simulink model "Model_2_1"  (R2024a)
settings: Solver=ode15s  StartTime=0.0  StopTime=100  FixedStep=0.0001  MaxStep=0.01  RelTol=1e-3  AbsTol=1e-3  EnableMultiTasking=on
model workspace (MATLAB code in the model file):
  | F_load_x= 0;   %[N]
  | F_load_y=-1e4; %[N]
  | 
  | d=0.01;   %[m]
  | l=1;      %[m]
  | L=l;      %[m] Node distance
  | H=l;      %[m] Node distance
  | Density=7800; %[kg/m^3]
  | E=210;   %[GPa]
  | G=79;    %[GPa]
  | bm=0.01; %[1/s] Default
  | bk=0.01; %[s] Default
  | 
  | b_rj=1; %[N*m*s/rad] Damp.Coef.Revolut joints
  | 
  | Size_frame=30; %[pixel]
undefined symbols (not defined in the file): F_x, F_y, X, Y, Z
libraries: sm_lib x173, nesl_utility x36, fl_lib x6, simulink x1
(part 1 of 5)
settings Model: NumberOfSteps=100000  Creator=Ing. Štefan Ondočko  LastModifiedBy=Ing. Štefan Ondočko
settings SolverCC: AutoScaleAbsTol=off  MaxZcPerStep=1
settings DataIOCC: LimitDataPoints=on  MaxDataPoints=10000  ReturnWorkspaceOutputs=off
settings OptimizationCC: ReuseModelBlockBuffer=off  LifeSpan=inf
settings DebuggingCC: UnconnectedInputMsg=warning  UnconnectedOutputMsg=warning  UnconnectedLineMsg=warning  AllowSymbolicDim=off  SubsystemReferenceDiagnosticForUnitTest=warning  SFUnexpectedBacktrackingDiag=warning  SFNoUnconditionalDefaultTransitionDiag=warning  SFExecutionAtInitializationDiag=none  ArithmeticOperatorsInVariantConditions=warning
settings ModelReferenceCC: EnableRefExpFcnMdlSchedulingChecks=on
settings SFSimCC: SimUseLocalCustomCode=off  CustomCodeUndefinedFunction=UseInterfaceOnly
settings RTWCC: RTWUseLocalCustomCode=off  GPUComputeCapability=3.5  DLArmComputeVersion=19.05
settings CodeAppCC: StateflowObjectComments=on
settings GRTTargetCC: TargetLangStandard=C89/C90 (ANSI)
settings ConfigComp: CovMetricSettings=dw  CovSaveCumulativeToWorkspaceVar=on  CovSaveSingleToWorkspaceVar=on  CovExternalEMLEnable=off  CovSFcnEnable=off
settings SimscapeCC: SimscapeLogType=all  SimscapeLogSimulationStatistics=on  SimscapeLogDataHistory=10000
settings ExplorerConfigSet: InternalSimMechanicsExplorerSettings="<ExplorerConfiguration><canonicalview>default</canonicalview><AnimationSetting><BasePlaybackSpeed>1.0</BasePlaybackSpeed><PlaybackSpeedFactor>2.0</PlaybackSpeedFactor></AnimationSetting><TilePanel><TileInfo><Tiles Columns=\"1\" Count=\"1\" Rows=\"1\"><Column Weight=\"1\"/><Row Weight=\"1\"/><Tile Height=\"1\" Width=\"1\" X=\"0\" Y=\"0\"/></Tiles></TileInfo><SceneInfo><SceneViewer><BGColor><R>1</R><G>1</G><B>1</B></BGColor><Camera><DoPerspective>off</DoPerspective><Position><X>1.34160017439744395</X><Y>2.43472426416735921</Y><Z>3.19868175252832421</Z></Position><Center><X>1.34160017439744395</X><Y>2.43472426416735921</Y><Z>1.1802899990698279e-08</Z></Center><Up><X>0</X><Y>1</Y><Z>-0</Z></Up><ViewLimDist>1</ViewLimDist><YLim>3.18022072065698147</YLim><XLim>1.97030216076793452</XLim></Camera></SceneViewer></SceneInfo></TilePanel><MechEditorPanel><Cameras/><GfxPanelCameraMap/><VideoCreator><PlaybackSpeedRatio>1.0</PlaybackSpeedRatio><FrameRate>30</FrameRate><VideoFormat>Motion JPEG AVI</VideoFormat><FrameSize>auto</FrameSize></VideoCreator></MechEditorPanel></ExplorerConfiguration>"

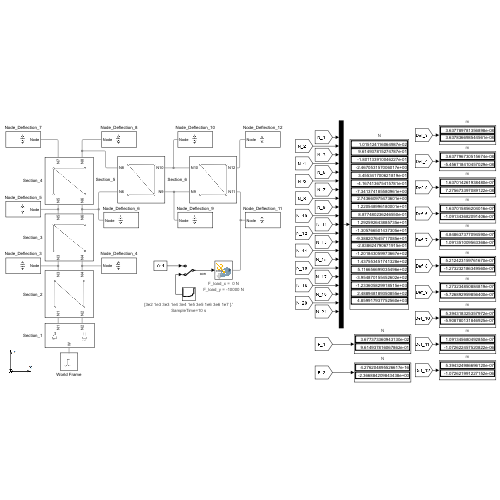
[thumbnail: Simulink's stored preview of the top-level diagram]
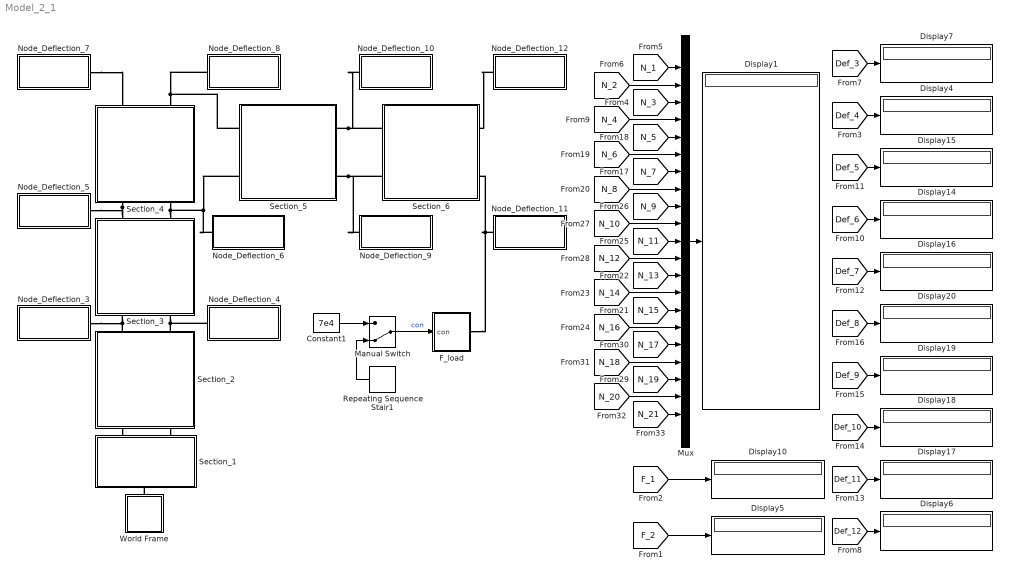
== system Model_2_1 ==
  Constant1 : Constant  Value=7e4
  Display{1,4..7,10,14..20} (13 alike) : Display
      Display1 settings: Description=N  AttributesFormatString=%<Description>  Format=long_e
      Display10 settings: Description=N  AttributesFormatString=%<Description>  Format=long_e
      Display14 settings: Description=m  AttributesFormatString=%<Description>  Format=long_e
      Display15 settings: Description=m  AttributesFormatString=%<Description>  Format=long_e
      Display16 settings: Description=m  AttributesFormatString=%<Description>  Format=long_e
      Display17 settings: Description=m  AttributesFormatString=%<Description>  Format=long_e
      Display18 settings: Description=m  AttributesFormatString=%<Description>  Format=long_e
      Display19 settings: Description=m  AttributesFormatString=%<Description>  Format=long_e
      Display20 settings: Description=m  AttributesFormatString=%<Description>  Format=long_e
      Display4 settings: Description=m  AttributesFormatString=%<Description>  Format=long_e
      Display5 settings: Description=N  AttributesFormatString=%<Description>  Format=long_e
      Display6 settings: Description=m  AttributesFormatString=%<Description>  Format=long_e
      Display7 settings: Description=m  AttributesFormatString=%<Description>  Format=long_e
  F_load : Subsystem  mask{Fx=F_load_x, Fy=F_load_y, F=norm([F_x F_y])}
      mask prompts: Fx "Load Fx (N)"; Fy "Load Fy (N)"; F "Load F (N)"
      settings: AttributesFormatString=|
      | %<Fx> =  0 N
      | %<Fy> = -10000 N
      mask Display: image('D:sila_F.png');
  Manual Switch : ManualSwitch  CurrentSetting=0
  Mux : Mux  Inputs=21
  Node_Deflection_10 : Subsystem
  Node_Deflection_11 : Subsystem
  Node_Deflection_12 : Subsystem
  Node_Deflection_3 : Subsystem
  Node_Deflection_4 : Subsystem
  Node_Deflection_5 : Subsystem
  Node_Deflection_6 : Subsystem
  Node_Deflection_7 : Subsystem
  Node_Deflection_8 : Subsystem
  Node_Deflection_9 : Subsystem
  Repeating Sequence Stair1 : simulink/Sources/Repeating Sequence Stair  OutValues=[3e2 1e3 3e3 1e4 3e4 1e5 3e5 1e6 3e6 1e7 ].'  tsamp=10  OutMin=[]  OutMax=[]  OutDataTypeStr=double  OutputDataTypeScalingMode=double  OutDataType=fixdt(0,8)  ConRadixGroup=Best Precision: Vector-wise  OutScaling=2^-12
      settings: AttributesFormatString=|
      | %<OutValues>
      | SampleTime=%<tsamp> s
  Section_1 : Subsystem
      settings: PortSchema="{\"entries\":[{\"content\":{\"sides\":[{\"content\":{},\"type\":\"ConnectorPlacement.EquallySpacedRectSide\",\"uuid\":\"639cab07-c461-4b38-814c-b2f66736f8dc\"},{\"content\":{\"side\":\"RIGHT\"},\"type\":\"ConnectorPlacement.EquallySpacedRectSide\",\"uuid\":\"511a9213-a72f-4349-881c-c7bf2be19ca2\"},{\"content\":{\"connectorIds\":[\"LConn1\"],\"side\":\"TOP\"},\"type\":\"ConnectorPlacement.EquallySpacedRectSide\",\"uuid\":\"5e8f2857-f7f3-429a-845e-93ee7ceff152\"},{\"content\":{\"connectorIds\":[\"RConn1\",\"RConn2\"],\"side\":\"BOTTOM\"},\"type\":\"ConnectorPlacement.EquallySpacedRectSide\",\"uuid\":\"39b416cf-f84e-45de-8d0c-fe880f5852f0\"}]},\"type\":\"ConnectorPlacement.EquallySpacedConnector\",\"uuid\":\"63df7647-7376-4d28-81b8-bff3ff006582\"}],\"packageUris\":[\"http://schema.mathworks.com/mf0/Connector/R2020b\"],\"version\":\"1.0\"}"
  Section_2 : Subsystem
      settings: PortSchema="{\"entries\":[{\"content\":{\"sides\":[{\"content\":{},\"type\":\"ConnectorPlacement.EquallySpacedRectSide\",\"uuid\":\"9852856a-cfaf-4274-b31b-57367341680d\"},{\"content\":{\"side\":\"RIGHT\"},\"type\":\"ConnectorPlacement.EquallySpacedRectSide\",\"uuid\":\"3ac774e0-1e79-4574-83fc-c3ad9c08ab46\"},{\"content\":{\"connectorIds\":[\"LConn1\",\"LConn2\"],\"side\":\"TOP\"},\"type\":\"ConnectorPlacement.EquallySpacedRectSide\",\"uuid\":\"0b881cdb-833a-4bc4-a75d-99faa647454f\"},{\"content\":{\"connectorIds\":[\"RConn1\",\"RConn2\"],\"side\":\"BOTTOM\"},\"type\":\"ConnectorPlacement.EquallySpacedRectSide\",\"uuid\":\"d5c54b3f-7996-4e81-879d-4e982bdffaf2\"}]},\"type\":\"ConnectorPlacement.EquallySpacedConnector\",\"uuid\":\"66ee5201-3e9b-4b60-9348-bbbcd71d5871\"}],\"packageUris\":[\"http://schema.mathworks.com/mf0/Connector/R2020b\"],\"version\":\"1.0\"}"
  Section_3 : Subsystem
      settings: PortSchema="{\"entries\":[{\"content\":{\"sides\":[{\"content\":{},\"type\":\"ConnectorPlacement.EquallySpacedRectSide\",\"uuid\":\"9852856a-cfaf-4274-b31b-57367341680d\"},{\"content\":{\"side\":\"RIGHT\"},\"type\":\"ConnectorPlacement.EquallySpacedRectSide\",\"uuid\":\"3ac774e0-1e79-4574-83fc-c3ad9c08ab46\"},{\"content\":{\"connectorIds\":[\"LConn1\",\"LConn2\"],\"side\":\"TOP\"},\"type\":\"ConnectorPlacement.EquallySpacedRectSide\",\"uuid\":\"0b881cdb-833a-4bc4-a75d-99faa647454f\"},{\"content\":{\"connectorIds\":[\"RConn1\",\"RConn2\"],\"side\":\"BOTTOM\"},\"type\":\"ConnectorPlacement.EquallySpacedRectSide\",\"uuid\":\"d5c54b3f-7996-4e81-879d-4e982bdffaf2\"}]},\"type\":\"ConnectorPlacement.EquallySpacedConnector\",\"uuid\":\"66ee5201-3e9b-4b60-9348-bbbcd71d5871\"}],\"packageUris\":[\"http://schema.mathworks.com/mf0/Connector/R2020b\"],\"version\":\"1.0\"}"
  Section_4 : Subsystem
      settings: PortSchema="{\"entries\":[{\"content\":{\"sides\":[{\"content\":{},\"type\":\"ConnectorPlacement.EquallySpacedRectSide\",\"uuid\":\"9852856a-cfaf-4274-b31b-57367341680d\"},{\"content\":{\"side\":\"RIGHT\"},\"type\":\"ConnectorPlacement.EquallySpacedRectSide\",\"uuid\":\"3ac774e0-1e79-4574-83fc-c3ad9c08ab46\"},{\"content\":{\"connectorIds\":[\"LConn1\",\"LConn2\"],\"side\":\"TOP\"},\"type\":\"ConnectorPlacement.EquallySpacedRectSide\",\"uuid\":\"0b881cdb-833a-4bc4-a75d-99faa647454f\"},{\"content\":{\"connectorIds\":[\"RConn1\",\"RConn2\"],\"side\":\"BOTTOM\"},\"type\":\"ConnectorPlacement.EquallySpacedRectSide\",\"uuid\":\"d5c54b3f-7996-4e81-879d-4e982bdffaf2\"}]},\"type\":\"ConnectorPlacement.EquallySpacedConnector\",\"uuid\":\"66ee5201-3e9b-4b60-9348-bbbcd71d5871\"}],\"packageUris\":[\"http://schema.mathworks.com/mf0/Connector/R2020b\"],\"version\":\"1.0\"}"
  Section_5 : Subsystem
      settings: PortSchema="{\"entries\":[{\"content\":{\"sides\":[{\"content\":{},\"type\":\"ConnectorPlacement.EquallySpacedRectSide\",\"uuid\":\"9852856a-cfaf-4274-b31b-57367341680d\"},{\"content\":{\"side\":\"RIGHT\"},\"type\":\"ConnectorPlacement.EquallySpacedRectSide\",\"uuid\":\"3ac774e0-1e79-4574-83fc-c3ad9c08ab46\"},{\"content\":{\"connectorIds\":[\"LConn1\",\"LConn2\"],\"side\":\"TOP\"},\"type\":\"ConnectorPlacement.EquallySpacedRectSide\",\"uuid\":\"0b881cdb-833a-4bc4-a75d-99faa647454f\"},{\"content\":{\"connectorIds\":[\"RConn1\",\"RConn2\"],\"side\":\"BOTTOM\"},\"type\":\"ConnectorPlacement.EquallySpacedRectSide\",\"uuid\":\"d5c54b3f-7996-4e81-879d-4e982bdffaf2\"}]},\"type\":\"ConnectorPlacement.EquallySpacedConnector\",\"uuid\":\"66ee5201-3e9b-4b60-9348-bbbcd71d5871\"}],\"packageUris\":[\"http://schema.mathworks.com/mf0/Connector/R2020b\"],\"version\":\"1.0\"}"
  Section_6 : Subsystem
      settings: PortSchema="{\"entries\":[{\"content\":{\"sides\":[{\"content\":{},\"type\":\"ConnectorPlacement.EquallySpacedRectSide\",\"uuid\":\"9852856a-cfaf-4274-b31b-57367341680d\"},{\"content\":{\"side\":\"RIGHT\"},\"type\":\"ConnectorPlacement.EquallySpacedRectSide\",\"uuid\":\"3ac774e0-1e79-4574-83fc-c3ad9c08ab46\"},{\"content\":{\"connectorIds\":[\"LConn1\",\"LConn2\"],\"side\":\"TOP\"},\"type\":\"ConnectorPlacement.EquallySpacedRectSide\",\"uuid\":\"0b881cdb-833a-4bc4-a75d-99faa647454f\"},{\"content\":{\"connectorIds\":[\"RConn1\",\"RConn2\"],\"side\":\"BOTTOM\"},\"type\":\"ConnectorPlacement.EquallySpacedRectSide\",\"uuid\":\"d5c54b3f-7996-4e81-879d-4e982bdffaf2\"}]},\"type\":\"ConnectorPlacement.EquallySpacedConnector\",\"uuid\":\"66ee5201-3e9b-4b60-9348-bbbcd71d5871\"}],\"packageUris\":[\"http://schema.mathworks.com/mf0/Connector/R2020b\"],\"version\":\"1.0\"}"
  World Frame : Subsystem
      settings: PortSchema="{\"entries\":[{\"content\":{\"sides\":[{\"content\":{},\"type\":\"ConnectorPlacement.EquallySpacedRectSide\",\"uuid\":\"6a8e21d3-b0b2-4758-a6c8-a7be5ecb73b9\"},{\"content\":{\"side\":\"RIGHT\"},\"type\":\"ConnectorPlacement.EquallySpacedRectSide\",\"uuid\":\"42798d98-bef9-4838-9935-056c1ef1235d\"},{\"content\":{\"connectorIds\":[\"LConn1\"],\"side\":\"TOP\"},\"type\":\"ConnectorPlacement.EquallySpacedRectSide\",\"uuid\":\"7c8f84cf-9fc0-4b00-b00b-766e511bcfac\"}]},\"type\":\"ConnectorPlacement.EquallySpacedConnector\",\"uuid\":\"93a5f294-2ff9-4ffa-a830-6e6e0d522148\"}],\"packageUris\":[\"http://schema.mathworks.com/mf0/Connector/R2020b\"],\"version\":\"1.0\"}"
  wires:
  Constant1/1 -> Manual Switch/1
  Manual Switch/1 -> F_load/1(con)  "con"
  [N_21] -> Mux/21
  Mux/1 -> Display1/1
  [N_20] -> Mux/20
  [N_18] -> Mux/18
  [N_16] -> Mux/16
  [N_12] -> Mux/12
  [N_5] -> Mux/5
  [N_10] -> Mux/10
  [N_4] -> Mux/4
  [N_2] -> Mux/2
  [N_17] -> Mux/17
  [N_19] -> Mux/19
  [N_15] -> Mux/15
  [Def_6] -> Display14/1
  [N_11] -> Mux/11
  [N_9] -> Mux/9
  [Def_9] -> Display19/1
  [N_7] -> Mux/7
  [Def_8] -> Display20/1
  [N_8] -> Mux/8
  [Def_11] -> Display17/1
  [N_1] -> Mux/1
  [N_14] -> Mux/14
  [Def_5] -> Display15/1
  [Def_7] -> Display16/1
  [N_3] -> Mux/3
  [N_6] -> Mux/6
  [Def_3] -> Display7/1
  [Def_10] -> Display18/1
  [N_13] -> Mux/13
  Repeating Sequence Stair1/1 -> Manual Switch/2
  [F_1] -> Display10/1
  [F_2] -> Display5/1
  [Def_12] -> Display6/1
  [Def_4] -> Display4/1
  connections:
  Node_Deflection_4/LConn1 -- Section_2/RConn2 -- Section_3/LConn2
  Node_Deflection_11/LConn1 -- F_load/RConn1 -- Section_6/LConn1
  Section_5/LConn1 -- Section_6/RConn1 -- Node_Deflection_9/LConn1
  Section_5/RConn1 -- Section_4/LConn2 -- Section_3/RConn2 -- Node_Deflection_6/LConn1
  Section_4/RConn2 -- Section_5/RConn2 -- Node_Deflection_8/LConn1
  Node_Deflection_3/LConn1 -- Section_2/RConn1 -- Section_3/LConn1
  Section_5/LConn2 -- Section_6/RConn2 -- Node_Deflection_10/LConn1
  Section_3/RConn1 -- Section_4/LConn1 -- Node_Deflection_5/LConn1
  Node_Deflection_12/LConn1 -- Section_6/LConn2
  Node_Deflection_7/LConn1 -- Section_4/RConn1
  World Frame/LConn1 -- Section_1/LConn1
  Section_2/LConn2 -- Section_1/RConn2
  Section_2/LConn1 -- Section_1/RConn1

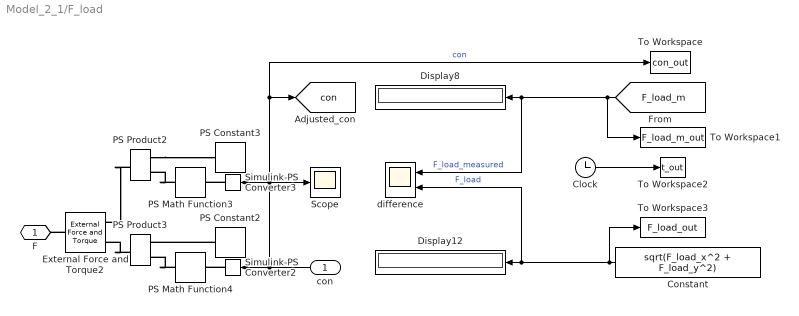
== system Model_2_1/F_load ==
  con : Inport
  Clock : Clock
  Constant : Constant  Value=sqrt(F_load_x^2 + F_load_y^2)
  Display12 : Display
      settings: Description=N  AttributesFormatString=%<Description>  Format=long_e
  Display8 : Display
      settings: Description=N  AttributesFormatString=%<Description>  Format=long_e
  External Force and Torque2 : sm_lib/Forces and Torques/External Force and Torque  EnableForceX=on  EnableForceY=on  EnableForceZ=off  EnableForce=off  ForceResolutionFrame=World  EnableTorqueX=off  EnableTorqueY=off  EnableTorqueZ=off  EnableTorque=off  TorqueResolutionFrame=AttachedFrame
  PS Constant2 : fl_lib/Physical Signals/Sources/PS Constant  constant=F_load_y
      settings: AttributesFormatString=%<constant>
  PS Constant3 : fl_lib/Physical Signals/Sources/PS Constant  constant=F_load_x
      settings: AttributesFormatString=%<constant>
  PS Math Function3 : fl_lib/Physical Signals/Functions/PS Math Function  fcn_choice=foundation.enum.math_function.reciprocal  v=1
  PS Math Function4 : fl_lib/Physical Signals/Functions/PS Math Function  fcn_choice=foundation.enum.math_function.reciprocal  v=1
  PS Product2 : fl_lib/Physical Signals/Functions/PS Product
  PS Product3 : fl_lib/Physical Signals/Functions/PS Product
  Scope : Scope
  Simulink-PS Converter2 : nesl_utility/Simulink-PS Converter  PhysicalDomain=network_engine_domain  SubClassName=ps_input  LeftPortType=input  RightPortType=output  PseudoPeriodic=off  Frequencies=[]  NoiseDistribution=none  NoiseParameters=[]  Unit=1  AffineConversion=off  FilteringAndDerivatives=provide  SimscapeFilterOrder=1  InputFilterTimeConstant=0.001  UdotUserProvided=0
  Simulink-PS Converter3 : nesl_utility/Simulink-PS Converter  PhysicalDomain=network_engine_domain  SubClassName=ps_input  LeftPortType=input  RightPortType=output  PseudoPeriodic=off  Frequencies=[]  NoiseDistribution=none  NoiseParameters=[]  Unit=1  AffineConversion=off  FilteringAndDerivatives=provide  SimscapeFilterOrder=1  InputFilterTimeConstant=0.001  UdotUserProvided=0
  To Workspace : ToWorkspace  VariableName=con_out  SampleTime=-1
  To Workspace1 : ToWorkspace  VariableName=F_load_m_out  SampleTime=-1
      settings: Decimation=3
  To Workspace2 : ToWorkspace  VariableName=t_out  SampleTime=-1
      settings: Decimation=3
  To Workspace3 : ToWorkspace  VariableName=F_load_out  SampleTime=-1
      settings: Decimation=3
  difference : Scope  NumInputPorts=2
  F : PMIOPort  Side=Right
  tag scope: con=global
  wires:
  [F_load_m] -> To Workspace1/1, difference/1, Display8/1  "F_load_measured"
  Constant/1 -> To Workspace3/1, Display12/1, difference/2  "F_load"
  Clock/1 -> To Workspace2/1
  con/1 -> To Workspace/1, [con], Scope/1, Simulink-PS Converter3/1, Simulink-PS Converter2/1  "con"
  connections:
  PS Math Function4/RConn1 -- PS Product3/LConn1
  Simulink-PS Converter2/RConn1 -- PS Math Function4/LConn1
  Simulink-PS Converter3/RConn1 -- PS Math Function3/LConn1
  PS Product2/LConn2 -- PS Constant3/RConn1
  PS Math Function3/RConn1 -- PS Product2/LConn1
  PS Constant2/RConn1 -- PS Product3/LConn2
  PS Product2/RConn1 -- External Force and Torque2/LConn1
  PS Product3/RConn1 -- External Force and Torque2/LConn2
  External Force and Torque2/RConn1 -- F/RConn1

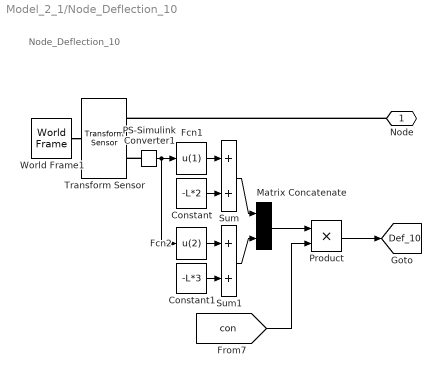
== system Model_2_1/Node_Deflection_10 ==
  note: Node_Deflection_10
  Constant : Constant  Value=-L*2
  Constant1 : Constant  Value=-L*3
  Fcn1 : Fcn  Expr=u(1)
  Fcn2 : Fcn  Expr=u(2)
  Matrix Concatenate : Concatenate  ConcatenateDimension=2
      settings: AttributesFormatString=%<Description>
  PS-Simulink Converter1 : nesl_utility/PS-Simulink Converter  PhysicalDomain=network_engine_domain  SubClassName=ps_output  LeftPortType=input  RightPortType=output  PseudoPeriodic=off  Frequencies=[]  VectorFormat=inherit  Unit=1  AffineConversion=off
  Product : Product
  Sum : Sum  Inputs=2
  Sum1 : Sum  Inputs=2
  Transform Sensor : sm_lib/Frames and Transforms/Transform Sensor  Description=|  MeasurementFrame=World  RotationSequence=XYX  SenseAngle=off  SenseAxis=off  SenseQ=off  SenseR=off  SenseRotationSequence=off  SenseOmegaX=off  SenseOmegaY=off  SenseOmegaZ=off  SenseOmega=off  SenseQDot=off  SenseRDot=off  SenseRotationSequenceDot=off  SenseAlphaX=off  SenseAlphaY=off  SenseAlphaZ=off  SenseAlpha=off  SenseQDDot=off  SenseRDDot=off  SenseX=off  SenseY=off  SenseZ=off  SenseXYZ=on  SenseRad=off  SenseAzim=off  SenseDist=off  SenseInc=off  SenseXDot=off  SenseYDot=off  SenseZDot=off  SenseXYZDot=off  SenseRadDot=off  SenseAzimDot=off  SenseDistDot=off  SenseIncDot=off  SenseXDDot=off  SenseYDDot=off  SenseZDDot=off  SenseXYZDDot=off  SenseRadDDot=off  SenseAzimDDot=off  SenseDistDDot=off  SenseIncDDot=off
      | Translation
      | [x, y, z]
      settings: AttributesFormatString=%<Description>
  World Frame1 : sm_lib/Frames and Transforms/World Frame
  Node : PMIOPort  Side=Left
  tag scope: Def_10=global
  wires:
  Fcn1/1 -> Sum/1
  Constant/1 -> Sum/2
  Sum/1 -> Matrix Concatenate/1
  Sum1/1 -> Matrix Concatenate/2
  Constant1/1 -> Sum1/2
  Fcn2/1 -> Sum1/1
  PS-Simulink Converter1/1 -> Fcn2/1, Fcn1/1
  Matrix Concatenate/1 -> Product/1
  [con] -> Product/2
  Product/1 -> [Def_10]
  connections:
  Node/RConn1 -- Transform Sensor/RConn1
  World Frame1/RConn1 -- Transform Sensor/LConn1
  PS-Simulink Converter1/LConn1 -- Transform Sensor/RConn2

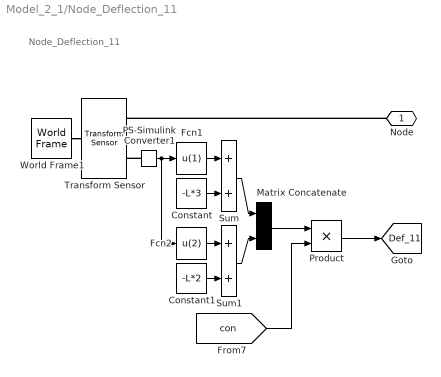
== system Model_2_1/Node_Deflection_11 ==
  note: Node_Deflection_11
  Constant : Constant  Value=-L*3
  Constant1 : Constant  Value=-L*2
  Fcn1 : Fcn  Expr=u(1)
  Fcn2 : Fcn  Expr=u(2)
  Matrix Concatenate : Concatenate  ConcatenateDimension=2
      settings: AttributesFormatString=%<Description>
  PS-Simulink Converter1 : nesl_utility/PS-Simulink Converter  PhysicalDomain=network_engine_domain  SubClassName=ps_output  LeftPortType=input  RightPortType=output  PseudoPeriodic=off  Frequencies=[]  VectorFormat=inherit  Unit=1  AffineConversion=off
  Product : Product
  Sum : Sum  Inputs=2
  Sum1 : Sum  Inputs=2
  Transform Sensor : sm_lib/Frames and Transforms/Transform Sensor  Description=|  MeasurementFrame=World  RotationSequence=XYX  SenseAngle=off  SenseAxis=off  SenseQ=off  SenseR=off  SenseRotationSequence=off  SenseOmegaX=off  SenseOmegaY=off  SenseOmegaZ=off  SenseOmega=off  SenseQDot=off  SenseRDot=off  SenseRotationSequenceDot=off  SenseAlphaX=off  SenseAlphaY=off  SenseAlphaZ=off  SenseAlpha=off  SenseQDDot=off  SenseRDDot=off  SenseX=off  SenseY=off  SenseZ=off  SenseXYZ=on  SenseRad=off  SenseAzim=off  SenseDist=off  SenseInc=off  SenseXDot=off  SenseYDot=off  SenseZDot=off  SenseXYZDot=off  SenseRadDot=off  SenseAzimDot=off  SenseDistDot=off  SenseIncDot=off  SenseXDDot=off  SenseYDDot=off  SenseZDDot=off  SenseXYZDDot=off  SenseRadDDot=off  SenseAzimDDot=off  SenseDistDDot=off  SenseIncDDot=off
      | Translation
      | [x, y, z]
      settings: AttributesFormatString=%<Description>
  World Frame1 : sm_lib/Frames and Transforms/World Frame
  Node : PMIOPort  Side=Left
  tag scope: Def_11=global
  wires:
  Product/1 -> [Def_11]
  [con] -> Product/2
  Matrix Concatenate/1 -> Product/1
  PS-Simulink Converter1/1 -> Fcn1/1, Fcn2/1
  Fcn2/1 -> Sum1/1
  Constant1/1 -> Sum1/2
  Sum1/1 -> Matrix Concatenate/2
  Sum/1 -> Matrix Concatenate/1
  Constant/1 -> Sum/2
  Fcn1/1 -> Sum/1
  connections:
  PS-Simulink Converter1/LConn1 -- Transform Sensor/RConn2
  World Frame1/RConn1 -- Transform Sensor/LConn1
  Node/RConn1 -- Transform Sensor/RConn1

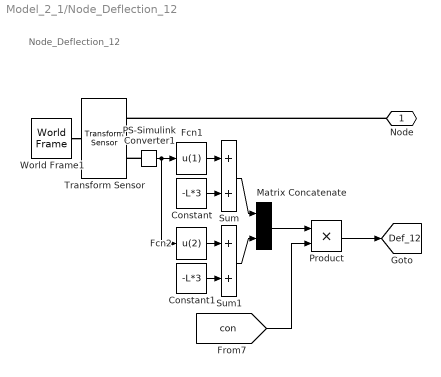
== system Model_2_1/Node_Deflection_12 ==
  note: Node_Deflection_12
  Constant : Constant  Value=-L*3
  Constant1 : Constant  Value=-L*3
  Fcn1 : Fcn  Expr=u(1)
  Fcn2 : Fcn  Expr=u(2)
  Matrix Concatenate : Concatenate  ConcatenateDimension=2
      settings: AttributesFormatString=%<Description>
  PS-Simulink Converter1 : nesl_utility/PS-Simulink Converter  PhysicalDomain=network_engine_domain  SubClassName=ps_output  LeftPortType=input  RightPortType=output  PseudoPeriodic=off  Frequencies=[]  VectorFormat=inherit  Unit=1  AffineConversion=off
  Product : Product
  Sum : Sum  Inputs=2
  Sum1 : Sum  Inputs=2
  Transform Sensor : sm_lib/Frames and Transforms/Transform Sensor  Description=|  MeasurementFrame=World  RotationSequence=XYX  SenseAngle=off  SenseAxis=off  SenseQ=off  SenseR=off  SenseRotationSequence=off  SenseOmegaX=off  SenseOmegaY=off  SenseOmegaZ=off  SenseOmega=off  SenseQDot=off  SenseRDot=off  SenseRotationSequenceDot=off  SenseAlphaX=off  SenseAlphaY=off  SenseAlphaZ=off  SenseAlpha=off  SenseQDDot=off  SenseRDDot=off  SenseX=off  SenseY=off  SenseZ=off  SenseXYZ=on  SenseRad=off  SenseAzim=off  SenseDist=off  SenseInc=off  SenseXDot=off  SenseYDot=off  SenseZDot=off  SenseXYZDot=off  SenseRadDot=off  SenseAzimDot=off  SenseDistDot=off  SenseIncDot=off  SenseXDDot=off  SenseYDDot=off  SenseZDDot=off  SenseXYZDDot=off  SenseRadDDot=off  SenseAzimDDot=off  SenseDistDDot=off  SenseIncDDot=off
      | Translation
      | [x, y, z]
      settings: AttributesFormatString=%<Description>
  World Frame1 : sm_lib/Frames and Transforms/World Frame
  Node : PMIOPort  Side=Left
  tag scope: Def_12=global
  wires:
  Fcn1/1 -> Sum/1
  Constant/1 -> Sum/2
  Sum/1 -> Matrix Concatenate/1
  Sum1/1 -> Matrix Concatenate/2
  Constant1/1 -> Sum1/2
  Fcn2/1 -> Sum1/1
  PS-Simulink Converter1/1 -> Fcn2/1, Fcn1/1
  Matrix Concatenate/1 -> Product/1
  [con] -> Product/2
  Product/1 -> [Def_12]
  connections:
  Node/RConn1 -- Transform Sensor/RConn1
  World Frame1/RConn1 -- Transform Sensor/LConn1
  PS-Simulink Converter1/LConn1 -- Transform Sensor/RConn2

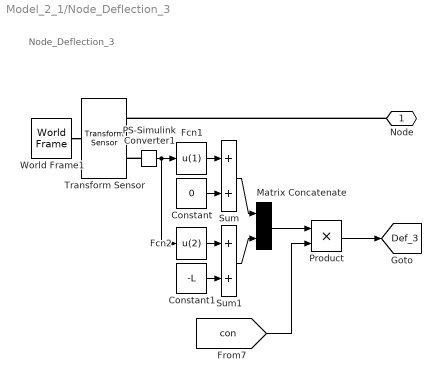
== system Model_2_1/Node_Deflection_3 ==
  note: Node_Deflection_3
  Constant : Constant  Value=0
  Constant1 : Constant  Value=-L
  Fcn1 : Fcn  Expr=u(1)
  Fcn2 : Fcn  Expr=u(2)
  Matrix Concatenate : Concatenate  ConcatenateDimension=2
      settings: AttributesFormatString=%<Description>
  PS-Simulink Converter1 : nesl_utility/PS-Simulink Converter  PhysicalDomain=network_engine_domain  SubClassName=ps_output  LeftPortType=input  RightPortType=output  PseudoPeriodic=off  Frequencies=[]  VectorFormat=inherit  Unit=1  AffineConversion=off
  Product : Product
  Sum : Sum  Inputs=2
  Sum1 : Sum  Inputs=2
  Transform Sensor : sm_lib/Frames and Transforms/Transform Sensor  Description=|  MeasurementFrame=World  RotationSequence=XYX  SenseAngle=off  SenseAxis=off  SenseQ=off  SenseR=off  SenseRotationSequence=off  SenseOmegaX=off  SenseOmegaY=off  SenseOmegaZ=off  SenseOmega=off  SenseQDot=off  SenseRDot=off  SenseRotationSequenceDot=off  SenseAlphaX=off  SenseAlphaY=off  SenseAlphaZ=off  SenseAlpha=off  SenseQDDot=off  SenseRDDot=off  SenseX=off  SenseY=off  SenseZ=off  SenseXYZ=on  SenseRad=off  SenseAzim=off  SenseDist=off  SenseInc=off  SenseXDot=off  SenseYDot=off  SenseZDot=off  SenseXYZDot=off  SenseRadDot=off  SenseAzimDot=off  SenseDistDot=off  SenseIncDot=off  SenseXDDot=off  SenseYDDot=off  SenseZDDot=off  SenseXYZDDot=off  SenseRadDDot=off  SenseAzimDDot=off  SenseDistDDot=off  SenseIncDDot=off
      | Translation
      | [x, y, z]
      settings: AttributesFormatString=%<Description>
  World Frame1 : sm_lib/Frames and Transforms/World Frame
  Node : PMIOPort  Side=Left
  tag scope: Def_3=global
  wires:
  Fcn1/1 -> Sum/1
  Constant/1 -> Sum/2
  Sum/1 -> Matrix Concatenate/1
  Sum1/1 -> Matrix Concatenate/2
  Constant1/1 -> Sum1/2
  Fcn2/1 -> Sum1/1
  PS-Simulink Converter1/1 -> Fcn2/1, Fcn1/1
  Matrix Concatenate/1 -> Product/1
  [con] -> Product/2
  Product/1 -> [Def_3]
  connections:
  Node/RConn1 -- Transform Sensor/RConn1
  World Frame1/RConn1 -- Transform Sensor/LConn1
  PS-Simulink Converter1/LConn1 -- Transform Sensor/RConn2

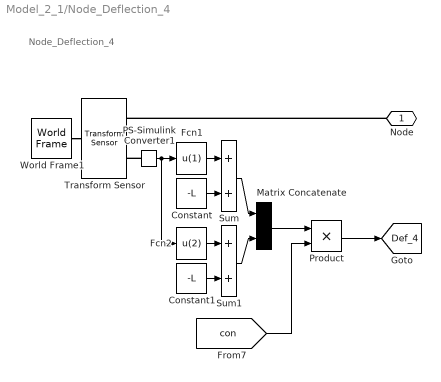
== system Model_2_1/Node_Deflection_4 ==
  note: Node_Deflection_4
  Constant : Constant  Value=-L
  Constant1 : Constant  Value=-L
  Fcn1 : Fcn  Expr=u(1)
  Fcn2 : Fcn  Expr=u(2)
  Matrix Concatenate : Concatenate  ConcatenateDimension=2
      settings: AttributesFormatString=%<Description>
  PS-Simulink Converter1 : nesl_utility/PS-Simulink Converter  PhysicalDomain=network_engine_domain  SubClassName=ps_output  LeftPortType=input  RightPortType=output  PseudoPeriodic=off  Frequencies=[]  VectorFormat=inherit  Unit=1  AffineConversion=off
  Product : Product
  Sum : Sum  Inputs=2
  Sum1 : Sum  Inputs=2
  Transform Sensor : sm_lib/Frames and Transforms/Transform Sensor  Description=|  MeasurementFrame=World  RotationSequence=XYX  SenseAngle=off  SenseAxis=off  SenseQ=off  SenseR=off  SenseRotationSequence=off  SenseOmegaX=off  SenseOmegaY=off  SenseOmegaZ=off  SenseOmega=off  SenseQDot=off  SenseRDot=off  SenseRotationSequenceDot=off  SenseAlphaX=off  SenseAlphaY=off  SenseAlphaZ=off  SenseAlpha=off  SenseQDDot=off  SenseRDDot=off  SenseX=off  SenseY=off  SenseZ=off  SenseXYZ=on  SenseRad=off  SenseAzim=off  SenseDist=off  SenseInc=off  SenseXDot=off  SenseYDot=off  SenseZDot=off  SenseXYZDot=off  SenseRadDot=off  SenseAzimDot=off  SenseDistDot=off  SenseIncDot=off  SenseXDDot=off  SenseYDDot=off  SenseZDDot=off  SenseXYZDDot=off  SenseRadDDot=off  SenseAzimDDot=off  SenseDistDDot=off  SenseIncDDot=off
      | Translation
      | [x, y, z]
      settings: AttributesFormatString=%<Description>
  World Frame1 : sm_lib/Frames and Transforms/World Frame
  Node : PMIOPort  Side=Left
  tag scope: Def_4=global
  wires:
  Fcn1/1 -> Sum/1
  Constant/1 -> Sum/2
  Sum/1 -> Matrix Concatenate/1
  Sum1/1 -> Matrix Concatenate/2
  Constant1/1 -> Sum1/2
  Fcn2/1 -> Sum1/1
  PS-Simulink Converter1/1 -> Fcn2/1, Fcn1/1
  Matrix Concatenate/1 -> Product/1
  [con] -> Product/2
  Product/1 -> [Def_4]
  connections:
  Node/RConn1 -- Transform Sensor/RConn1
  World Frame1/RConn1 -- Transform Sensor/LConn1
  PS-Simulink Converter1/LConn1 -- Transform Sensor/RConn2

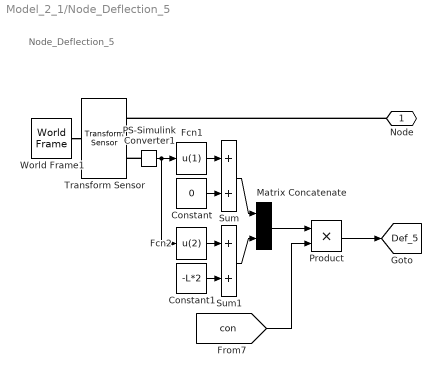
== system Model_2_1/Node_Deflection_5 ==
  note: Node_Deflection_5
  Constant : Constant  Value=0
  Constant1 : Constant  Value=-L*2
  Fcn1 : Fcn  Expr=u(1)
  Fcn2 : Fcn  Expr=u(2)
  Matrix Concatenate : Concatenate  ConcatenateDimension=2
      settings: AttributesFormatString=%<Description>
  PS-Simulink Converter1 : nesl_utility/PS-Simulink Converter  PhysicalDomain=network_engine_domain  SubClassName=ps_output  LeftPortType=input  RightPortType=output  PseudoPeriodic=off  Frequencies=[]  VectorFormat=inherit  Unit=1  AffineConversion=off
  Product : Product
  Sum : Sum  Inputs=2
  Sum1 : Sum  Inputs=2
  Transform Sensor : sm_lib/Frames and Transforms/Transform Sensor  Description=|  MeasurementFrame=World  RotationSequence=XYX  SenseAngle=off  SenseAxis=off  SenseQ=off  SenseR=off  SenseRotationSequence=off  SenseOmegaX=off  SenseOmegaY=off  SenseOmegaZ=off  SenseOmega=off  SenseQDot=off  SenseRDot=off  SenseRotationSequenceDot=off  SenseAlphaX=off  SenseAlphaY=off  SenseAlphaZ=off  SenseAlpha=off  SenseQDDot=off  SenseRDDot=off  SenseX=off  SenseY=off  SenseZ=off  SenseXYZ=on  SenseRad=off  SenseAzim=off  SenseDist=off  SenseInc=off  SenseXDot=off  SenseYDot=off  SenseZDot=off  SenseXYZDot=off  SenseRadDot=off  SenseAzimDot=off  SenseDistDot=off  SenseIncDot=off  SenseXDDot=off  SenseYDDot=off  SenseZDDot=off  SenseXYZDDot=off  SenseRadDDot=off  SenseAzimDDot=off  SenseDistDDot=off  SenseIncDDot=off
      | Translation
      | [x, y, z]
      settings: AttributesFormatString=%<Description>
  World Frame1 : sm_lib/Frames and Transforms/World Frame
  Node : PMIOPort  Side=Left
  tag scope: Def_5=global
  wires:
  Product/1 -> [Def_5]
  [con] -> Product/2
  Matrix Concatenate/1 -> Product/1
  PS-Simulink Converter1/1 -> Fcn1/1, Fcn2/1
  Fcn2/1 -> Sum1/1
  Constant1/1 -> Sum1/2
  Sum1/1 -> Matrix Concatenate/2
  Sum/1 -> Matrix Concatenate/1
  Constant/1 -> Sum/2
  Fcn1/1 -> Sum/1
  connections:
  PS-Simulink Converter1/LConn1 -- Transform Sensor/RConn2
  World Frame1/RConn1 -- Transform Sensor/LConn1
  Node/RConn1 -- Transform Sensor/RConn1

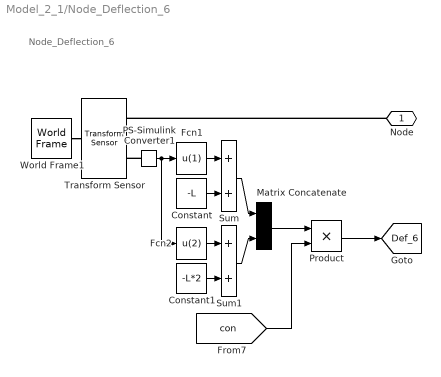
== system Model_2_1/Node_Deflection_6 ==
  note: Node_Deflection_6
  Constant : Constant  Value=-L
  Constant1 : Constant  Value=-L*2
  Fcn1 : Fcn  Expr=u(1)
  Fcn2 : Fcn  Expr=u(2)
  Matrix Concatenate : Concatenate  ConcatenateDimension=2
      settings: AttributesFormatString=%<Description>
  PS-Simulink Converter1 : nesl_utility/PS-Simulink Converter  PhysicalDomain=network_engine_domain  SubClassName=ps_output  LeftPortType=input  RightPortType=output  PseudoPeriodic=off  Frequencies=[]  VectorFormat=inherit  Unit=1  AffineConversion=off
  Product : Product
  Sum : Sum  Inputs=2
  Sum1 : Sum  Inputs=2
  Transform Sensor : sm_lib/Frames and Transforms/Transform Sensor  Description=|  MeasurementFrame=World  RotationSequence=XYX  SenseAngle=off  SenseAxis=off  SenseQ=off  SenseR=off  SenseRotationSequence=off  SenseOmegaX=off  SenseOmegaY=off  SenseOmegaZ=off  SenseOmega=off  SenseQDot=off  SenseRDot=off  SenseRotationSequenceDot=off  SenseAlphaX=off  SenseAlphaY=off  SenseAlphaZ=off  SenseAlpha=off  SenseQDDot=off  SenseRDDot=off  SenseX=off  SenseY=off  SenseZ=off  SenseXYZ=on  SenseRad=off  SenseAzim=off  SenseDist=off  SenseInc=off  SenseXDot=off  SenseYDot=off  SenseZDot=off  SenseXYZDot=off  SenseRadDot=off  SenseAzimDot=off  SenseDistDot=off  SenseIncDot=off  SenseXDDot=off  SenseYDDot=off  SenseZDDot=off  SenseXYZDDot=off  SenseRadDDot=off  SenseAzimDDot=off  SenseDistDDot=off  SenseIncDDot=off
      | Translation
      | [x, y, z]
      settings: AttributesFormatString=%<Description>
  World Frame1 : sm_lib/Frames and Transforms/World Frame
  Node : PMIOPort  Side=Left
  tag scope: Def_6=global
  wires:
  Product/1 -> [Def_6]
  [con] -> Product/2
  Matrix Concatenate/1 -> Product/1
  PS-Simulink Converter1/1 -> Fcn1/1, Fcn2/1
  Fcn2/1 -> Sum1/1
  Constant1/1 -> Sum1/2
  Sum1/1 -> Matrix Concatenate/2
  Sum/1 -> Matrix Concatenate/1
  Constant/1 -> Sum/2
  Fcn1/1 -> Sum/1
  connections:
  PS-Simulink Converter1/LConn1 -- Transform Sensor/RConn2
  World Frame1/RConn1 -- Transform Sensor/LConn1
  Node/RConn1 -- Transform Sensor/RConn1

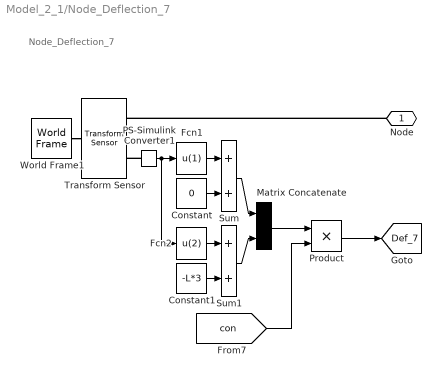
== system Model_2_1/Node_Deflection_7 ==
  note: Node_Deflection_7
  Constant : Constant  Value=0
  Constant1 : Constant  Value=-L*3
  Fcn1 : Fcn  Expr=u(1)
  Fcn2 : Fcn  Expr=u(2)
  Matrix Concatenate : Concatenate  ConcatenateDimension=2
      settings: AttributesFormatString=%<Description>
  PS-Simulink Converter1 : nesl_utility/PS-Simulink Converter  PhysicalDomain=network_engine_domain  SubClassName=ps_output  LeftPortType=input  RightPortType=output  PseudoPeriodic=off  Frequencies=[]  VectorFormat=inherit  Unit=1  AffineConversion=off
  Product : Product
  Sum : Sum  Inputs=2
  Sum1 : Sum  Inputs=2
  Transform Sensor : sm_lib/Frames and Transforms/Transform Sensor  Description=|  MeasurementFrame=World  RotationSequence=XYX  SenseAngle=off  SenseAxis=off  SenseQ=off  SenseR=off  SenseRotationSequence=off  SenseOmegaX=off  SenseOmegaY=off  SenseOmegaZ=off  SenseOmega=off  SenseQDot=off  SenseRDot=off  SenseRotationSequenceDot=off  SenseAlphaX=off  SenseAlphaY=off  SenseAlphaZ=off  SenseAlpha=off  SenseQDDot=off  SenseRDDot=off  SenseX=off  SenseY=off  SenseZ=off  SenseXYZ=on  SenseRad=off  SenseAzim=off  SenseDist=off  SenseInc=off  SenseXDot=off  SenseYDot=off  SenseZDot=off  SenseXYZDot=off  SenseRadDot=off  SenseAzimDot=off  SenseDistDot=off  SenseIncDot=off  SenseXDDot=off  SenseYDDot=off  SenseZDDot=off  SenseXYZDDot=off  SenseRadDDot=off  SenseAzimDDot=off  SenseDistDDot=off  SenseIncDDot=off
      | Translation
      | [x, y, z]
      settings: AttributesFormatString=%<Description>
  World Frame1 : sm_lib/Frames and Transforms/World Frame
  Node : PMIOPort  Side=Left
  tag scope: Def_7=global
  wires:
  Fcn1/1 -> Sum/1
  Constant/1 -> Sum/2
  Sum/1 -> Matrix Concatenate/1
  Sum1/1 -> Matrix Concatenate/2
  Constant1/1 -> Sum1/2
  Fcn2/1 -> Sum1/1
  PS-Simulink Converter1/1 -> Fcn2/1, Fcn1/1
  Matrix Concatenate/1 -> Product/1
  [con] -> Product/2
  Product/1 -> [Def_7]
  connections:
  Node/RConn1 -- Transform Sensor/RConn1
  World Frame1/RConn1 -- Transform Sensor/LConn1
  PS-Simulink Converter1/LConn1 -- Transform Sensor/RConn2

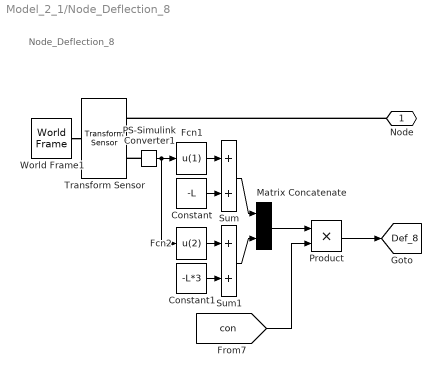
== system Model_2_1/Node_Deflection_8 ==
  note: Node_Deflection_8
  Constant : Constant  Value=-L
  Constant1 : Constant  Value=-L*3
  Fcn1 : Fcn  Expr=u(1)
  Fcn2 : Fcn  Expr=u(2)
  Matrix Concatenate : Concatenate  ConcatenateDimension=2
      settings: AttributesFormatString=%<Description>
  PS-Simulink Converter1 : nesl_utility/PS-Simulink Converter  PhysicalDomain=network_engine_domain  SubClassName=ps_output  LeftPortType=input  RightPortType=output  PseudoPeriodic=off  Frequencies=[]  VectorFormat=inherit  Unit=1  AffineConversion=off
  Product : Product
  Sum : Sum  Inputs=2
  Sum1 : Sum  Inputs=2
  Transform Sensor : sm_lib/Frames and Transforms/Transform Sensor  Description=|  MeasurementFrame=World  RotationSequence=XYX  SenseAngle=off  SenseAxis=off  SenseQ=off  SenseR=off  SenseRotationSequence=off  SenseOmegaX=off  SenseOmegaY=off  SenseOmegaZ=off  SenseOmega=off  SenseQDot=off  SenseRDot=off  SenseRotationSequenceDot=off  SenseAlphaX=off  SenseAlphaY=off  SenseAlphaZ=off  SenseAlpha=off  SenseQDDot=off  SenseRDDot=off  SenseX=off  SenseY=off  SenseZ=off  SenseXYZ=on  SenseRad=off  SenseAzim=off  SenseDist=off  SenseInc=off  SenseXDot=off  SenseYDot=off  SenseZDot=off  SenseXYZDot=off  SenseRadDot=off  SenseAzimDot=off  SenseDistDot=off  SenseIncDot=off  SenseXDDot=off  SenseYDDot=off  SenseZDDot=off  SenseXYZDDot=off  SenseRadDDot=off  SenseAzimDDot=off  SenseDistDDot=off  SenseIncDDot=off
      | Translation
      | [x, y, z]
      settings: AttributesFormatString=%<Description>
  World Frame1 : sm_lib/Frames and Transforms/World Frame
  Node : PMIOPort  Side=Left
  tag scope: Def_8=global
  wires:
  Fcn1/1 -> Sum/1
  Constant/1 -> Sum/2
  Sum/1 -> Matrix Concatenate/1
  Sum1/1 -> Matrix Concatenate/2
  Constant1/1 -> Sum1/2
  Fcn2/1 -> Sum1/1
  PS-Simulink Converter1/1 -> Fcn2/1, Fcn1/1
  Matrix Concatenate/1 -> Product/1
  [con] -> Product/2
  Product/1 -> [Def_8]
  connections:
  Node/RConn1 -- Transform Sensor/RConn1
  World Frame1/RConn1 -- Transform Sensor/LConn1
  PS-Simulink Converter1/LConn1 -- Transform Sensor/RConn2

== system Model_2_1/Node_Deflection_9 ==
  note: Node_Deflection_9
  Constant : Constant  Value=-L*2
  Constant1 : Constant  Value=-L*2
  Fcn1 : Fcn  Expr=u(1)
  Fcn2 : Fcn  Expr=u(2)
  Matrix Concatenate : Concatenate  ConcatenateDimension=2
      settings: AttributesFormatString=%<Description>
  PS-Simulink Converter1 : nesl_utility/PS-Simulink Converter  PhysicalDomain=network_engine_domain  SubClassName=ps_output  LeftPortType=input  RightPortType=output  PseudoPeriodic=off  Frequencies=[]  VectorFormat=inherit  Unit=1  AffineConversion=off
  Product : Product
  Sum : Sum  Inputs=2
  Sum1 : Sum  Inputs=2
  Transform Sensor : sm_lib/Frames and Transforms/Transform Sensor  Description=|  MeasurementFrame=World  RotationSequence=XYX  SenseAngle=off  SenseAxis=off  SenseQ=off  SenseR=off  SenseRotationSequence=off  SenseOmegaX=off  SenseOmegaY=off  SenseOmegaZ=off  SenseOmega=off  SenseQDot=off  SenseRDot=off  SenseRotationSequenceDot=off  SenseAlphaX=off  SenseAlphaY=off  SenseAlphaZ=off  SenseAlpha=off  SenseQDDot=off  SenseRDDot=off  SenseX=off  SenseY=off  SenseZ=off  SenseXYZ=on  SenseRad=off  SenseAzim=off  SenseDist=off  SenseInc=off  SenseXDot=off  SenseYDot=off  SenseZDot=off  SenseXYZDot=off  SenseRadDot=off  SenseAzimDot=off  SenseDistDot=off  SenseIncDot=off  SenseXDDot=off  SenseYDDot=off  SenseZDDot=off  SenseXYZDDot=off  SenseRadDDot=off  SenseAzimDDot=off  SenseDistDDot=off  SenseIncDDot=off
      | Translation
      | [x, y, z]
      settings: AttributesFormatString=%<Description>
  World Frame1 : sm_lib/Frames and Transforms/World Frame
  Node : PMIOPort  Side=Left
  tag scope: Def_9=global
  wires:
  Product/1 -> [Def_9]
  [con] -> Product/2
  Matrix Concatenate/1 -> Product/1
  PS-Simulink Converter1/1 -> Fcn1/1, Fcn2/1
  Fcn2/1 -> Sum1/1
  Constant1/1 -> Sum1/2
  Sum1/1 -> Matrix Concatenate/2
  Sum/1 -> Matrix Concatenate/1
  Constant/1 -> Sum/2
  Fcn1/1 -> Sum/1
  connections:
  PS-Simulink Converter1/LConn1 -- Transform Sensor/RConn2
  World Frame1/RConn1 -- Transform Sensor/LConn1
  Node/RConn1 -- Transform Sensor/RConn1

== system Model_2_1/Section_1 ==
  Beam_1 : Subsystem
  Node_1 : Subsystem
      settings: PortSchema="{\"entries\":[{\"content\":{\"sides\":[{\"content\":{},\"type\":\"ConnectorPlacement.EquallySpacedRectSide\",\"uuid\":\"aca6bf7c-dcc8-4964-93f9-4a1fe43793ee\"},{\"content\":{\"connectorIds\":[\"RConn1\"],\"side\":\"RIGHT\"},\"type\":\"ConnectorPlacement.EquallySpacedRectSide\",\"uuid\":\"dab82db3-710a-4609-884f-38beebf819d8\"},{\"content\":{\"connectorIds\":[\"LConn1\"],\"side\":\"TOP\"},\"type\":\"ConnectorPlacement.EquallySpacedRectSide\",\"uuid\":\"19f47c76-519b-4e1a-8863-c1336a5f880a\"}]},\"type\":\"ConnectorPlacement.EquallySpacedConnector\",\"uuid\":\"649caf1b-1885-49fa-b181-e591fe1aead3\"}],\"packageUris\":[\"http://schema.mathworks.com/mf0/Connector/R2020b\"],\"version\":\"1.0\"}"
  Node_2 : Subsystem
      settings: PortSchema="{\"entries\":[{\"content\":{\"sides\":[{\"content\":{},\"type\":\"ConnectorPlacement.EquallySpacedRectSide\",\"uuid\":\"e4796b0d-43bb-40a6-b678-1855539de64a\"},{\"content\":{\"connectorIds\":[\"RConn1\"],\"side\":\"RIGHT\"},\"type\":\"ConnectorPlacement.EquallySpacedRectSide\",\"uuid\":\"30db7710-eb1e-4112-bf9f-d5c657b92c9d\"},{\"content\":{\"connectorIds\":[\"LConn1\"],\"side\":\"TOP\"},\"type\":\"ConnectorPlacement.EquallySpacedRectSide\",\"uuid\":\"9a38070c-035d-4b3b-9197-abd4c8b486d2\"},{\"content\":{\"side\":\"BOTTOM\"},\"type\":\"ConnectorPlacement.EquallySpacedRectSide\",\"uuid\":\"e9dd2cf3-dbcb-47d4-bd9b-dfaab0188d3c\"}]},\"type\":\"ConnectorPlacement.EquallySpacedConnector\",\"uuid\":\"963d3d3c-e3eb-4536-b22c-5a90b7423a96\"}],\"packageUris\":[\"http://schema.mathworks.com/mf0/Connector/R2020b\"],\"version\":\"1.0\"}"
  Rigid Transform : sm_lib/Frames and Transforms/Rigid Transform  RotationMethod=StandardAxis  FollAlignAxisA=+X  BaseAlignAxisA=+Y  FollAlignAxisB=+Y  BaseAlignAxisB=+Z  RotationStandardAxis=+Z  RotationAngle=pi/2  RotationAngleUnits=rad  RotationArbitraryAxis=[0 0 1]  RotationSequenceAxes=FollowerAxes  RotationSequence=XYX  RotationSequenceAngles=[0 0 0]  RotationSequenceAnglesUnits=deg  RotationMatrix=[1 0 0;0 1 0;0 0 1]  Quaternion=[1 0 0 0]  TranslationMethod=None  TranslationCartesianOffset=[0 0 0]  TranslationCartesianOffsetUnits=m  TranslationStandardAxis=+Z  TranslationStandardOffset=0  TranslationStandardOffsetUnits=m  TranslationROffset=0  TranslationROffsetUnits=m  TranslationThetaOffset=0  TranslationThetaOffsetUnits=deg  TranslationZOffset=0  TranslationZOffsetUnits=m
      settings: AttributesFormatString=%<RotationAngle>
  W : PMIOPort  Side=Left
  N1 : PMIOPort  Port=2  Side=Right
  N2 : PMIOPort  Port=3  Side=Right
  connections:
  Node_1/LConn1 -- Node_2/LConn1 -- W/RConn1
  Rigid Transform/LConn1 -- Beam_1/LConn1 -- Node_1/RConn1
  Beam_1/RConn1 -- Node_2/RConn1 -- N2/RConn1
  N1/RConn1 -- Rigid Transform/RConn1

== system Model_2_1/Section_2 ==
  Beam_2 : Subsystem
  Beam_3 : Subsystem
  Beam_4 : Subsystem
  Beam_5 : Subsystem
  Node_1 : Subsystem
      settings: PortSchema="{\"entries\":[{\"content\":{\"sides\":[{\"content\":{},\"type\":\"ConnectorPlacement.EquallySpacedRectSide\",\"uuid\":\"8515b1c5-3545-41e3-b118-13ff900d4b29\"},{\"content\":{\"side\":\"RIGHT\"},\"type\":\"ConnectorPlacement.EquallySpacedRectSide\",\"uuid\":\"a9ef51d2-c79d-4a36-af02-f81a35fa3e5b\"},{\"content\":{\"connectorIds\":[\"LConn1\"],\"side\":\"TOP\"},\"type\":\"ConnectorPlacement.EquallySpacedRectSide\",\"uuid\":\"f027515f-1122-484c-940f-7281e35c2be1\"},{\"content\":{\"connectorIds\":[\"RConn1\"],\"side\":\"BOTTOM\"},\"type\":\"ConnectorPlacement.EquallySpacedRectSide\",\"uuid\":\"53053ac7-4cfd-4112-8186-1f6ff745e7f3\"}]},\"type\":\"ConnectorPlacement.EquallySpacedConnector\",\"uuid\":\"2ea7d68c-970c-4c50-bafe-de90d81019d0\"}],\"packageUris\":[\"http://schema.mathworks.com/mf0/Connector/R2020b\"],\"version\":\"1.0\"}"
  Node_2 : Subsystem
      settings: PortSchema="{\"entries\":[{\"content\":{\"sides\":[{\"content\":{},\"type\":\"ConnectorPlacement.EquallySpacedRectSide\",\"uuid\":\"01fbe943-d1b3-448b-a169-5bcf29c0e4f2\"},{\"content\":{\"side\":\"RIGHT\"},\"type\":\"ConnectorPlacement.EquallySpacedRectSide\",\"uuid\":\"10891364-c263-49ec-ba31-f6a87e2d8ee4\"},{\"content\":{\"connectorIds\":[\"LConn1\"],\"side\":\"TOP\"},\"type\":\"ConnectorPlacement.EquallySpacedRectSide\",\"uuid\":\"7927076a-ca63-430c-95f4-6324d7761717\"},{\"content\":{\"connectorIds\":[\"RConn1\",\"RConn2\"],\"side\":\"BOTTOM\"},\"type\":\"ConnectorPlacement.EquallySpacedRectSide\",\"uuid\":\"ea4595de-581c-4702-b786-ba2f35ddf078\"}]},\"type\":\"ConnectorPlacement.EquallySpacedConnector\",\"uuid\":\"450777ed-a8dd-4d83-a6b2-860fbce0f68b\"}],\"packageUris\":[\"http://schema.mathworks.com/mf0/Connector/R2020b\"],\"version\":\"1.0\"}"
  Node_3 : Subsystem
      settings: PortSchema="{\"entries\":[{\"content\":{\"sides\":[{\"content\":{},\"type\":\"ConnectorPlacement.EquallySpacedRectSide\",\"uuid\":\"8515b1c5-3545-41e3-b118-13ff900d4b29\"},{\"content\":{\"connectorIds\":[\"RConn1\",\"RConn2\"],\"side\":\"RIGHT\"},\"type\":\"ConnectorPlacement.EquallySpacedRectSide\",\"uuid\":\"a9ef51d2-c79d-4a36-af02-f81a35fa3e5b\"},{\"content\":{\"connectorIds\":[\"LConn1\"],\"side\":\"TOP\"},\"type\":\"ConnectorPlacement.EquallySpacedRectSide\",\"uuid\":\"f027515f-1122-484c-940f-7281e35c2be1\"},{\"content\":{\"connectorIds\":[\"RConn3\"],\"side\":\"BOTTOM\"},\"type\":\"ConnectorPlacement.EquallySpacedRectSide\",\"uuid\":\"53053ac7-4cfd-4112-8186-1f6ff745e7f3\"}]},\"type\":\"ConnectorPlacement.EquallySpacedConnector\",\"uuid\":\"2ea7d68c-970c-4c50-bafe-de90d81019d0\"}],\"packageUris\":[\"http://schema.mathworks.com/mf0/Connector/R2020b\"],\"version\":\"1.0\"}"
  Node_4 : Subsystem
      settings: PortSchema="{\"entries\":[{\"content\":{\"sides\":[{\"content\":{\"connectorIds\":[\"LConn1\"]},\"type\":\"ConnectorPlacement.EquallySpacedRectSide\",\"uuid\":\"01fbe943-d1b3-448b-a169-5bcf29c0e4f2\"},{\"content\":{\"side\":\"RIGHT\"},\"type\":\"ConnectorPlacement.EquallySpacedRectSide\",\"uuid\":\"10891364-c263-49ec-ba31-f6a87e2d8ee4\"},{\"content\":{\"connectorIds\":[\"LConn2\"],\"side\":\"TOP\"},\"type\":\"ConnectorPlacement.EquallySpacedRectSide\",\"uuid\":\"7927076a-ca63-430c-95f4-6324d7761717\"},{\"content\":{\"connectorIds\":[\"RConn1\"],\"side\":\"BOTTOM\"},\"type\":\"ConnectorPlacement.EquallySpacedRectSide\",\"uuid\":\"ea4595de-581c-4702-b786-ba2f35ddf078\"}]},\"type\":\"ConnectorPlacement.EquallySpacedConnector\",\"uuid\":\"450777ed-a8dd-4d83-a6b2-860fbce0f68b\"}],\"packageUris\":[\"http://schema.mathworks.com/mf0/Connector/R2020b\"],\"version\":\"1.0\"}"
  N1 : PMIOPort  Side=Left
  N2 : PMIOPort  Port=2  Side=Left
  N3 : PMIOPort  Port=3  Side=Right
  N4 : PMIOPort  Port=4  Side=Right
  connections:
  N2/RConn1 -- Node_2/LConn1
  Node_4/RConn1 -- N4/RConn1
  N3/RConn1 -- Node_3/RConn3
  Node_4/LConn1 -- Beam_5/RConn1
  Node_3/RConn2 -- Beam_5/LConn1
  Beam_4/RConn1 -- Node_4/LConn2
  Node_2/RConn1 -- Beam_3/RConn1
  Node_1/LConn1 -- N1/RConn1
  Beam_2/RConn1 -- Node_3/LConn1
  Node_3/RConn1 -- Beam_3/LConn1
  Beam_4/LConn1 -- Node_2/RConn2
  Node_1/RConn1 -- Beam_2/LConn1

== system Model_2_1/Section_3 ==
  Beam_6 : Subsystem
  Beam_7 : Subsystem
  Beam_8 : Subsystem
  Beam_9 : Subsystem
  Node_3 : Subsystem
      settings: PortSchema="{\"entries\":[{\"content\":{\"sides\":[{\"content\":{},\"type\":\"ConnectorPlacement.EquallySpacedRectSide\",\"uuid\":\"8515b1c5-3545-41e3-b118-13ff900d4b29\"},{\"content\":{\"side\":\"RIGHT\"},\"type\":\"ConnectorPlacement.EquallySpacedRectSide\",\"uuid\":\"a9ef51d2-c79d-4a36-af02-f81a35fa3e5b\"},{\"content\":{\"connectorIds\":[\"LConn1\"],\"side\":\"TOP\"},\"type\":\"ConnectorPlacement.EquallySpacedRectSide\",\"uuid\":\"f027515f-1122-484c-940f-7281e35c2be1\"},{\"content\":{\"connectorIds\":[\"RConn1\"],\"side\":\"BOTTOM\"},\"type\":\"ConnectorPlacement.EquallySpacedRectSide\",\"uuid\":\"53053ac7-4cfd-4112-8186-1f6ff745e7f3\"}]},\"type\":\"ConnectorPlacement.EquallySpacedConnector\",\"uuid\":\"2ea7d68c-970c-4c50-bafe-de90d81019d0\"}],\"packageUris\":[\"http://schema.mathworks.com/mf0/Connector/R2020b\"],\"version\":\"1.0\"}"
  Node_4 : Subsystem
      settings: PortSchema="{\"entries\":[{\"content\":{\"sides\":[{\"content\":{},\"type\":\"ConnectorPlacement.EquallySpacedRectSide\",\"uuid\":\"01fbe943-d1b3-448b-a169-5bcf29c0e4f2\"},{\"content\":{\"side\":\"RIGHT\"},\"type\":\"ConnectorPlacement.EquallySpacedRectSide\",\"uuid\":\"10891364-c263-49ec-ba31-f6a87e2d8ee4\"},{\"content\":{\"connectorIds\":[\"LConn1\"],\"side\":\"TOP\"},\"type\":\"ConnectorPlacement.EquallySpacedRectSide\",\"uuid\":\"7927076a-ca63-430c-95f4-6324d7761717\"},{\"content\":{\"connectorIds\":[\"RConn1\",\"RConn2\"],\"side\":\"BOTTOM\"},\"type\":\"ConnectorPlacement.EquallySpacedRectSide\",\"uuid\":\"ea4595de-581c-4702-b786-ba2f35ddf078\"}]},\"type\":\"ConnectorPlacement.EquallySpacedConnector\",\"uuid\":\"450777ed-a8dd-4d83-a6b2-860fbce0f68b\"}],\"packageUris\":[\"http://schema.mathworks.com/mf0/Connector/R2020b\"],\"version\":\"1.0\"}"
  Node_5 : Subsystem
      settings: PortSchema="{\"entries\":[{\"content\":{\"sides\":[{\"content\":{},\"type\":\"ConnectorPlacement.EquallySpacedRectSide\",\"uuid\":\"8515b1c5-3545-41e3-b118-13ff900d4b29\"},{\"content\":{\"connectorIds\":[\"RConn1\",\"RConn2\"],\"side\":\"RIGHT\"},\"type\":\"ConnectorPlacement.EquallySpacedRectSide\",\"uuid\":\"a9ef51d2-c79d-4a36-af02-f81a35fa3e5b\"},{\"content\":{\"connectorIds\":[\"LConn1\"],\"side\":\"TOP\"},\"type\":\"ConnectorPlacement.EquallySpacedRectSide\",\"uuid\":\"f027515f-1122-484c-940f-7281e35c2be1\"},{\"content\":{\"connectorIds\":[\"RConn3\"],\"side\":\"BOTTOM\"},\"type\":\"ConnectorPlacement.EquallySpacedRectSide\",\"uuid\":\"53053ac7-4cfd-4112-8186-1f6ff745e7f3\"}]},\"type\":\"ConnectorPlacement.EquallySpacedConnector\",\"uuid\":\"2ea7d68c-970c-4c50-bafe-de90d81019d0\"}],\"packageUris\":[\"http://schema.mathworks.com/mf0/Connector/R2020b\"],\"version\":\"1.0\"}"
  Node_6 : Subsystem
      settings: PortSchema="{\"entries\":[{\"content\":{\"sides\":[{\"content\":{\"connectorIds\":[\"LConn1\"]},\"type\":\"ConnectorPlacement.EquallySpacedRectSide\",\"uuid\":\"01fbe943-d1b3-448b-a169-5bcf29c0e4f2\"},{\"content\":{\"side\":\"RIGHT\"},\"type\":\"ConnectorPlacement.EquallySpacedRectSide\",\"uuid\":\"10891364-c263-49ec-ba31-f6a87e2d8ee4\"},{\"content\":{\"connectorIds\":[\"LConn2\"],\"side\":\"TOP\"},\"type\":\"ConnectorPlacement.EquallySpacedRectSide\",\"uuid\":\"7927076a-ca63-430c-95f4-6324d7761717\"},{\"content\":{\"connectorIds\":[\"RConn1\"],\"side\":\"BOTTOM\"},\"type\":\"ConnectorPlacement.EquallySpacedRectSide\",\"uuid\":\"ea4595de-581c-4702-b786-ba2f35ddf078\"}]},\"type\":\"ConnectorPlacement.EquallySpacedConnector\",\"uuid\":\"450777ed-a8dd-4d83-a6b2-860fbce0f68b\"}],\"packageUris\":[\"http://schema.mathworks.com/mf0/Connector/R2020b\"],\"version\":\"1.0\"}"
  N3 : PMIOPort  Side=Left
  N4 : PMIOPort  Port=2  Side=Left
  N5 : PMIOPort  Port=3  Side=Right
  N6 : PMIOPort  Port=4  Side=Right
  connections:
  Beam_6/LConn1 -- Node_3/RConn1
  Beam_8/LConn1 -- Node_4/RConn2
  Node_5/RConn1 -- Beam_7/LConn1
  Beam_6/RConn1 -- Node_5/LConn1
  Node_3/LConn1 -- N3/RConn1
  Node_4/RConn1 -- Beam_7/RConn1
  Beam_8/RConn1 -- Node_6/LConn2
  Node_5/RConn2 -- Beam_9/LConn1
  Node_6/LConn1 -- Beam_9/RConn1
  N5/RConn1 -- Node_5/RConn3
  Node_6/RConn1 -- N6/RConn1
  N4/RConn1 -- Node_4/LConn1
